simulink model "AdaptiveMPPT"  (R2017a)
settings: Solver=ode45  StartTime=0.0  StopTime=.02  RelTol=1e-3  EnableMultiTasking=on
libraries: powerlib x12, simulink x2, powerlib_extras x1, re_lib x1
settings Model: Creator=user  LastModifiedBy=acer
settings DataIOCC: LimitDataPoints=on  SaveFormat=Array
settings OptimizationCC: LifeSpan=inf
settings DebuggingCC: SFUnexpectedBacktrackingDiag=warning  SFNoUnconditionalDefaultTransitionDiag=warning  SFExecutionAtInitializationDiag=none
settings HardwareCC: ProdBitPerPointer=32  ProdBitPerSizeT=32  ProdBitPerPtrDiffT=32  ProdLargestAtomicFloat=None  ProdIntDivRoundTo=Undefined  ProdEndianess=Unspecified  ProdWordSize=32  ProdHWDeviceType=32-bit Generic
settings ModelReferenceCC: PropagateSignalLabelsOutOfModel=off
settings GRTTargetCC: TargetLangStandard=C89/C90 (ANSI)  GeneratePreprocessorConditionals=Disable all
settings ConfigComp: CovMetricSettings=dw  CovHtmlReporting=on  CovSaveCumulativeToWorkspaceVar=on  CovSaveSingleToWorkspaceVar=on  CovExternalEMLEnable=off

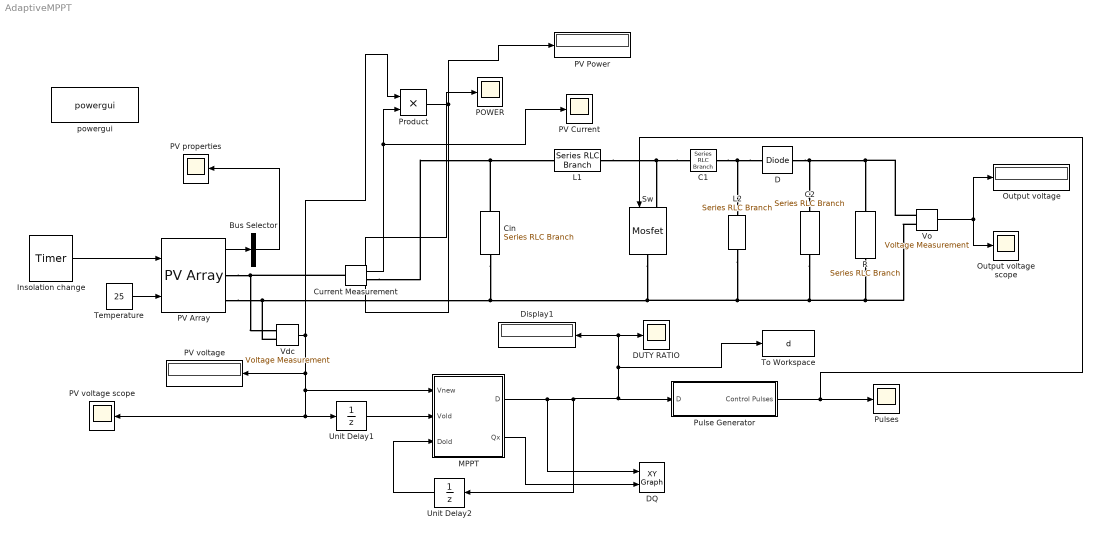
== system AdaptiveMPPT ==
  Bus Selector : BusSelector  OutputSignals=V_PV,I_PV  OutputAsBus=on
  C1 : powerlib/Elements/Series RLC Branch  LConnTagsString=__new0  RConnTagsString=__new0  BranchType=C  Resistance=100  Inductance=1e-3  SetiL0=off  InitialCurrent=0  Capacitance=20e-6  Setx0=off  InitialVoltage=0  Measurements=None
  C2 : powerlib/Elements/Series RLC Branch  LConnTagsString=__new0  RConnTagsString=__new0  BranchType=C  Resistance=1  Inductance=1e-3  SetiL0=off  InitialCurrent=0  Capacitance=150e-6  Setx0=off  InitialVoltage=0  Measurements=None
  Cin : powerlib/Elements/Series RLC Branch  LConnTagsString=__new0  RConnTagsString=__new0  BranchType=C  Resistance=1  Inductance=1e-3  SetiL0=off  InitialCurrent=0  Capacitance=100e-6  Setx0=off  InitialVoltage=0  Measurements=None
  Current Measurement : powerlib/Measurements/Current Measurement  PhasorSimulation=off  OutputType=Complex  PSBequivalent=0
  D : powerlib/Power Electronics/Diode  Ron=0.001  Lon=0  Vf=.05  IC=0  UseSnubber=off  Rs=500  Cs=250e-9  Measurements=off
  DQ : simulink/Sinks/XY Graph  xmin=0  xmax=.02  ymin=0  ymax=3  st=.0001
  DUTY RATIO : Scope
  Display1 : Display
  Insolation change : powerlib_extras/Control  Blocks/Timer  t="[0  .01]"  e="[270   480]"
  L1 : powerlib/Elements/Series RLC Branch  LConnTagsString=__new0  RConnTagsString=__new0  BranchType=L  Resistance=1  Inductance=90e-6  SetiL0=off  InitialCurrent=0  Capacitance=1e-6  Setx0=off  InitialVoltage=0  Measurements=None
  L2 : powerlib/Elements/Series RLC Branch  LConnTagsString=__new0  RConnTagsString=__new0  BranchType=L  Resistance=1  Inductance=90e-6  SetiL0=off  InitialCurrent=0  Capacitance=1e-6  Setx0=off  InitialVoltage=0  Measurements=None
  MPPT : MATLAB Function  TreatAsAtomicUnit=on
  Output voltage : Display
  Output voltage scope : Scope
  POWER : Scope
  PV Array : re_lib/Solar/PV Array  Npar=9  Nser=4  PlotType=one module @ 25 deg.C & specified irradiances  S_vec=[270 480]  Temp_C_vec="[ 45 25  ]"  ModuleName=User-defined  PlotWhenSelected=on  Pm=20.1544  Ncell=36  Voc=21.17  Isc=1.26  Vm=17.08  Im=1.18  beta_Voc_pc=-0.2941  alpha_Isc_pc=0.0681  beta_Voc=-0.062261  alpha_Isc=0.00085806  IL=1.2621  I0=3.4157e-12  nI=0.85997  Rsh=849.2491  Rs=1.4265  BAL=on  Tc=1e-6  Tfilter=2e-5
  PV Current : Scope
  PV Power : Display
  PV properties : Scope
  PV voltage : Display
  PV voltage scope : Scope
  Product : Product
  Pulse Generator : Subsystem  mask{F=50e3}
      mask prompts: F "Carrier Frequency"
  Pulses : Scope
  R : powerlib/Elements/Series RLC Branch  LConnTagsString=__new0  RConnTagsString=__new0  BranchType=R  Resistance=10  Inductance=1e-3  SetiL0=off  InitialCurrent=0  Capacitance=1e-6  Setx0=off  InitialVoltage=0  Measurements=None
  Sw : powerlib/Power Electronics/Mosfet  Ron=0.1  Lon=0  Rd=0.01  Vfd=0  IC=0  Rs=1e5  Cs=inf  Measurements=off
  Temperature : Constant  Value=25  VectorParams1D=off  SampleTime=2e-5
  To Workspace : ToWorkspace  VariableName=d  SaveFormat=Timeseries  SampleTime=-1
  Unit Delay1 : UnitDelay  SampleTime=.0001
  Unit Delay2 : UnitDelay  SampleTime=.0001
  "Vdc " : powerlib/Measurements/Voltage Measurement  Tag=PoWeRsYsTeMmEaSuReMeNt  PhasorSimulation=off  OutputType=Magnitude  PSBequivalent=0
  Vo : powerlib/Measurements/Voltage Measurement  PhasorSimulation=off  OutputType=Complex  PSBequivalent=0
  powergui : powerlib/powergui  Priority=1  SimulationMode=Discrete  SampleTime=50e-6  frequency=50  Iterations=50  frequencyindice=0  Pbase=100e6  ErrMax=1e-4  UnitsV=kV  UnitsW=MW  buscounter=0  FunctionMessages=off  echomessages=off  EnableUseOfTLC=off  CurrentSourceSwitches=off  DisableSnubberDevices=off  DisableRonSwitches=off  DisableVfSwitches=on  DisplayEquations=off  SolverType=Tustin/Backward Euler (TBE)  Interpol=off  ExternalGateDelay=off  methode=off  Ts=0  x0status=blocks  SPID=on  SwTol=0  HookPort=off  RestoreLinks=warning  ResistiveCurrentMeasurement=off  Frange=[0:2:500]  Ylog=off  Xlog=on  ShowGrid=off  save=off  variable=ZData  structure=0  ZoomFFT=on  StartTime=0.0  cycles=1  DisplayStyle=1  fundamental=60  FreqAxis=off  MaxFrequency=1000  frequencyindicesteady=1  RmsSteady=1  display=off
  wires:
  PV Array/1 -> Bus Selector/1
  Vo/1 -> Output voltage scope/1, Output voltage/1
  MPPT/1(D) -> DQ/1, Unit Delay2/1, To Workspace/1, DUTY RATIO/1, Display1/1, Pulse Generator/1(D)
  Pulse Generator/1(Control Pulses) -> Sw/1, Pulses/1
  Bus Selector/1 -> PV properties/1
  Unit Delay2/1 -> MPPT/3(Dold)
  Temperature/1 -> PV Array/2
  "Vdc "/1 -> PV voltage/1, PV voltage scope/1, Unit Delay1/1, MPPT/1(Vnew), Product/1
  MPPT/2(Qx) -> DQ/2
  Unit Delay1/1 -> MPPT/2(Vold)
  Product/1 -> PV Power/1, POWER/1
  Current Measurement/1 -> PV Current/1, Product/2
  Insolation change/1 -> PV Array/1
  connections:
  Vo/LConn2 -- R/RConn1 -- C2/RConn1 -- L2/RConn1 -- Cin/RConn1 -- PV Array/RConn2 -- "Vdc "/LConn2 -- Sw/RConn1
  C1/LConn1 -- Sw/LConn1 -- L1/RConn1
  C2/LConn1 -- D/RConn1 -- Vo/LConn1 -- R/LConn1
  D/LConn1 -- L2/LConn1 -- C1/RConn1
  Current Measurement/RConn1 -- Cin/LConn1 -- L1/LConn1
  PV Array/RConn1 -- "Vdc "/LConn1 -- Current Measurement/LConn1

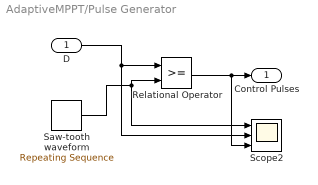
== system AdaptiveMPPT/Pulse Generator ==
  D : Inport
  Relational Operator : RelationalOperator  OutDataTypeStr=boolean  RndMeth=Nearest
  Saw-tooth waveform : simulink/Sources/Repeating Sequence  rep_seq_t=[0 0.5 1]/F  rep_seq_y=[0 1 0]
  Scope2 : Scope  NumInputPorts=3
  Control Pulses : Outport
  wires:
  Saw-tooth waveform/1 -> Relational Operator/2, Scope2/1
  Relational Operator/1 -> Scope2/3, Control Pulses/1
  D/1 -> Relational Operator/1, Scope2/2

== matlab function AdaptiveMPPT/MPPT ==
  data: Vnew input; Vold input; Dold input; D output; Qx output
%Calculate Q
function [D,Qx] = MPPT(Vnew,Vold,Dold)
M1=.0001;
M2=.01;
disp('Vnew');
disp(Vnew);
disp('Vold');
disp(Vold);
disp('Dold');
disp(Dold);
%Dmax = .409416581
% Qth = (.409416581*(1-.409416581)*.0003))+(17*.0001)
Qth = .001772538393;
Vdel =Vnew - Vold;
Ddel = .0001;
Qx=((1-Dold)*Vdel)+(Vnew*Ddel);
Q=abs(Qx);
if (Q>=Qth)
    disp('large');
    dD = M1*Q;
else
    disp('small');
    dD = M2*Q;
end
disp(Q);
if (Qx>0)
    D = Dold+dD;
else if (Qx<0)
        D = Dold-dD;
    else
        D = Dold;
    end
end
